simulink model "generator_library"  (R2019b)
settings: Solver=VariableStepAuto  StartTime=0.0  StopTime=10.0  RelTol=1e-3
undefined symbols (not defined in the file or in its folder): dataSim, dyn, Fnom, g, genTpd0, genTppd0, genTppq0, genTpq0, genXd, genXl, genXpd, genXppd, genXppq, genXpq, genXq, ifd, l, p, sys, vt
libraries: powerlib x27, simulink x10, powerlib_meascontrol x5, GenLib x2
settings Model: Creator=gdudgeon  LastModifiedBy=gdudgeon
settings SFSimCC: CustomCodeUndefinedFunction=UseInterfaceOnly

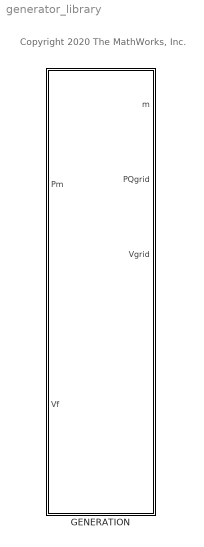
== system generator_library ==
  note: Copyright 2020 The MathWorks, Inc.
  GENERATION : Subsystem  VariantControlMode=Label  Variant=on  LabelModeActiveChoice=Variant2
      settings: AttributesFormatString=%<BlockChoice>

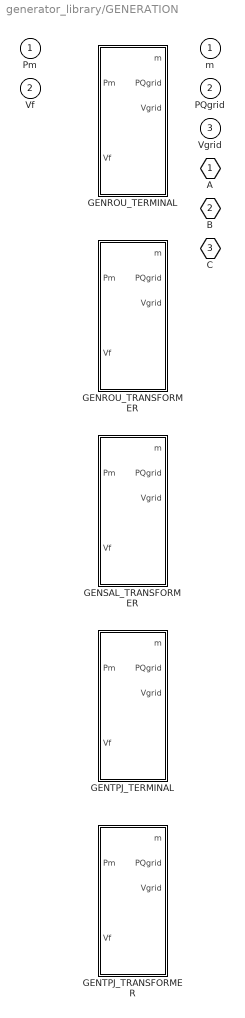
== system generator_library/GENERATION ==
  Pm : Inport
  Vf : Inport  Port=2
  GENROU_TERMINAL : Subsystem  VariantControl=Variant1  mask{g=sys.GENERATOR(1), p=dyn.genrou_31923_COLUSGT1}
      mask prompts: g "Generator Parameters"; p "Dynamic Parameters"
      mask DialogControl DescGroupVar Prompt: GENROU_TRANSFORMER
  GENROU_TRANSFORMER : Subsystem  VariantControl=Variant2  mask{g=sys.GENERATOR(2), t=sys.TRANSFORMER, p=dyn.genrou_102_GAS}
      mask prompts: g "Generator Parameters"; t "Transformer Parameters"; p "Dynamic Parameters"
      mask DialogControl DescGroupVar Prompt: GENROU_TRANSFORMER
  GENSAL_TRANSFORMER : Subsystem  VariantControl=Variant3  mask{g=sys.GENERATOR(2), t=sys.TRANSFORMER, p=dyn.gentpj_102_HYDRO}
      mask prompts: g "Generator Parameters"; t "Transformer Parameters"; p "Dynamic Parameters"
      mask DialogControl DescGroupVar Prompt: GENSAL_TRANSFORMER
  GENTPJ_TERMINAL : Subsystem  VariantControl=Variant4  mask{g=g, t=t, p=p}
      mask prompts: g "Generator Parameters"; t "Transformer Parameters"; p "Dynamic Parameters"
      mask DialogControl DescGroupVar Prompt: GENTPJ_TRANSFORMER
  GENTPJ_TRANSFORMER : Subsystem  VariantControl=Variant5  mask{g=sys.GENERATOR(2), t=sys.TRANSFORMER, p=dyn.gentpj_102_HYDRO}
      mask prompts: g "Generator Parameters"; t "Transformer Parameters"; p "Dynamic Parameters"
      mask DialogControl DescGroupVar Prompt: GENTPJ_TRANSFORMER
  A : PMIOPort  Side=Right
  B : PMIOPort  Port=2  Side=Right
  C : PMIOPort  Port=3  Side=Right
  m : Outport  VectorParamsAs1DForOutWhenUnconnected=off
  PQgrid : Outport  Port=2  VectorParamsAs1DForOutWhenUnconnected=off
  Vgrid : Outport  Port=3  VectorParamsAs1DForOutWhenUnconnected=off

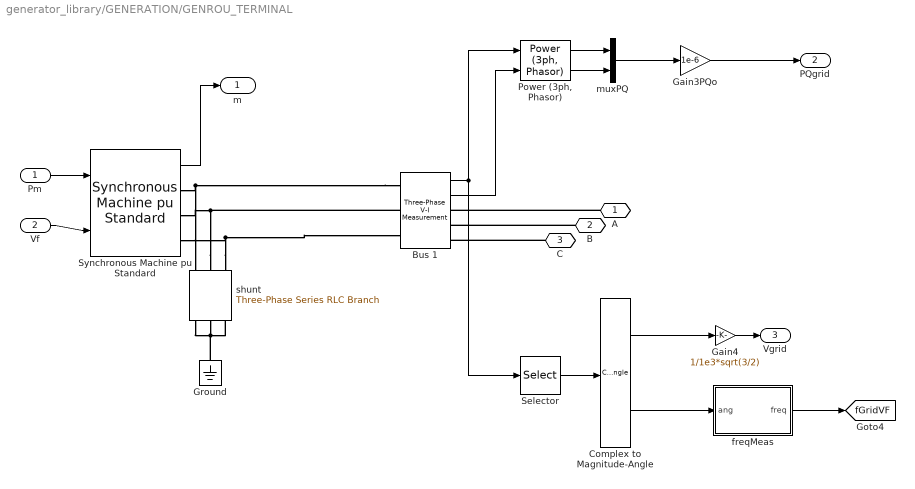
== system generator_library/GENERATION/GENROU_TERMINAL ==
  Pm : Inport
  Vf : Inport  Port=2
  Bus 1 : powerlib/Measurements/Three-Phase V-I Measurement  VoltageMeasurement=phase-to-ground  SetLabelV=off  LabelV=Vabc  Vpu=off  VpuLL=off  CurrentMeasurement=yes  SetLabelI=off  LabelI=Iabc  Ipu=off  Pbase=100e6  Vbase=500e3  OutputType=Complex  PhasorSimulation=on  PSBequivalent=0
      settings: SourceProductName=Simscape Electrical
  Complex to Magnitude-Angle : ComplexToMagnitudeAngle
  Gain3PQo : Gain  Gain=1e-6
  Gain4 : Gain  Gain=1/1e3*sqrt(3/2)
  Ground : powerlib/Elements/Ground  LConnTagsString=a
      settings: SourceProductName=Simscape Electrical
  "Power (3ph, Phasor)" : powerlib_meascontrol/Measurements/Power (3ph, Phasor)
      settings: SourceProductName=Simscape Electrical  SourceProductBaseCode=PS
  Selector : Selector  InputPortWidth=3  IndexOptions=Index vector (dialog)  Indices=1  OutputSizes=1
  Synchronous Machine pu Standard : powerlib/Machines/Synchronous Machine pu Standard  PresetModel=No  MechanicalLoad=Mechanical power Pm  ShowDetailedParameters=on  RotorType=Round  Units=per unit standard parameters  MeasurementBus=off  NominalParameters=[g.MBASE*1e6 g.BUSV*1e3 60]  Reactances1=[p.ld p.lpd p.lppd p.lq p.lpq p.lppd p.ll-0.01]  Reactances2=[ genXd genXpd genXppd genXq genXpq genXppq genXl]  dAxisTimeConstants=Open-circuit  qAxisTimeConstants=Open-circuit  TimeConstants1="[ 4.4849  0.0681  0.1  ]"  TimeConstants2=[p.tpdo p.tppdo p.tpqo p.tppqo]  TimeConstants3="[  4.49  0.0681  0.0513  ]"  TimeConstants4=[ 8.0, 0.03, 0.3371, 0.0295 ]  TimeConstants5=[ 1.01, 0.053, 0.1 ]  TimeConstants6=[ 1.3201, 0.023, 1.0, 0.07 ]  TimeConstants7=[genTpd0 genTppd0 genTpq0 genTppq0]  TimeConstants8=[genTpd0 genTppd0 genTpq0 genTppq0]  StatorResistance=p.ra  Mechanical=[p.h p.d 2]  PolePairs=2  InitialConditions=[0 -89.4885 0.00587296 0.00587296 0.00587296 0 -120 120 1.00004]  SetSaturation=on  Saturation=[ifd; vt]  LoadFlowParameters=[2 0 0 0 0]  TsPowergui=0  TsBlock=-1  IterativeModel=Trapezoidal non iterative  IterativeDiscreteModel=Trapezoidal non iterative  BusType=PV  Pref=0  Qref=0  Qmin=-inf  Qmax=inf  PLF=0  QLF=0
      settings: SourceProductName=Simscape Electrical
  freqMeas : Subsystem
  muxPQ : Mux  Inputs=2
  shunt : powerlib/Elements/Three-Phase Series RLC Branch  LConnTagsString=A|B|C  RConnTagsString=A|B|C  BranchType=R  Resistance=1e6  Inductance=0.0025  Capacitance=0  Measurements=None
      settings: SourceProductName=Simscape Electrical
  A : PMIOPort  Side=Right
  B : PMIOPort  Port=2  Side=Right
  C : PMIOPort  Port=3  Side=Right
  m : Outport  VectorParamsAs1DForOutWhenUnconnected=off
  PQgrid : Outport  Port=2  VectorParamsAs1DForOutWhenUnconnected=off
  Vgrid : Outport  Port=3  VectorParamsAs1DForOutWhenUnconnected=off
  tag scope: fGridVF=global
  wires:
  muxPQ/1 -> Gain3PQo/1
  Bus 1/1 -> Selector/1, "Power (3ph, Phasor)"/1
  Bus 1/2 -> "Power (3ph, Phasor)"/2
  "Power (3ph, Phasor)"/1 -> muxPQ/1
  Pm/1 -> Synchronous Machine pu Standard/1
  Complex to Magnitude-Angle/1 -> Gain4/1
  Vf/1 -> Synchronous Machine pu Standard/2
  Gain3PQo/1 -> PQgrid/1
  Gain4/1 -> Vgrid/1
  "Power (3ph, Phasor)"/2 -> muxPQ/2
  Synchronous Machine pu Standard/1 -> m/1
  Selector/1 -> Complex to Magnitude-Angle/1
  Complex to Magnitude-Angle/2 -> freqMeas/1(ang)
  freqMeas/1(freq) -> [fGridVF]
  connections:
  shunt/LConn3 -- Bus 1/LConn3 -- Synchronous Machine pu Standard/RConn3
  Bus 1/LConn1 -- shunt/LConn1 -- Synchronous Machine pu Standard/RConn1
  shunt/LConn2 -- Bus 1/LConn2 -- Synchronous Machine pu Standard/RConn2
  A/RConn1 -- Bus 1/RConn1
  B/RConn1 -- Bus 1/RConn2
  C/RConn1 -- Bus 1/RConn3
  shunt/RConn1 -- Ground/LConn1 -- shunt/RConn2 -- shunt/RConn3

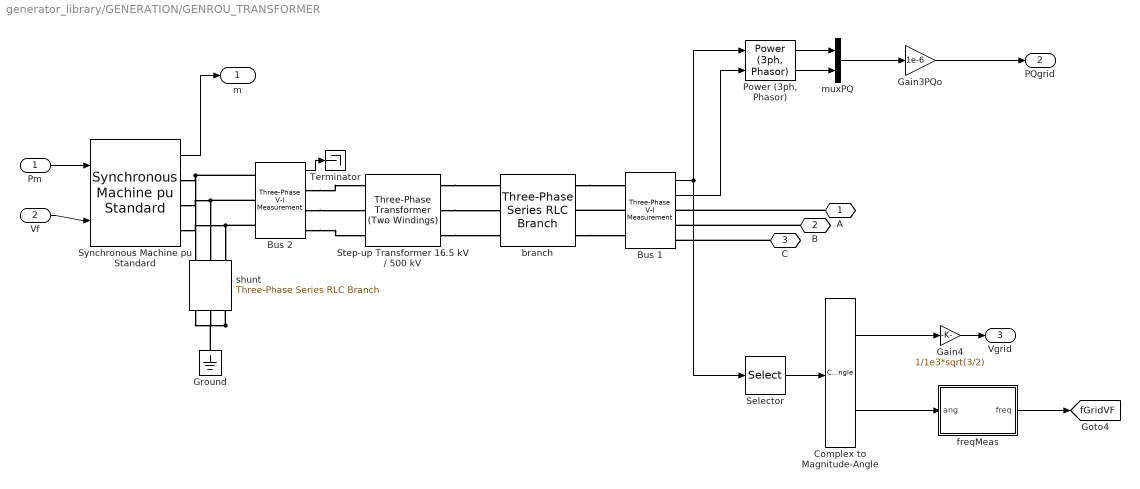
== system generator_library/GENERATION/GENROU_TRANSFORMER ==
  Pm : Inport
  Vf : Inport  Port=2
  Bus 1 : powerlib/Measurements/Three-Phase V-I Measurement  VoltageMeasurement=phase-to-ground  SetLabelV=off  LabelV=Vabc  Vpu=off  VpuLL=off  CurrentMeasurement=yes  SetLabelI=off  LabelI=Iabc  Ipu=off  Pbase=100e6  Vbase=500e3  OutputType=Complex  PhasorSimulation=on  PSBequivalent=0
      settings: SourceProductName=Simscape Electrical
  Bus 2 : powerlib/Measurements/Three-Phase V-I Measurement  VoltageMeasurement=phase-to-ground  SetLabelV=off  LabelV=Vabc  Vpu=off  VpuLL=off  CurrentMeasurement=no  SetLabelI=off  LabelI=Iabc  Ipu=off  Pbase=100e6  Vbase=500e3  OutputType=Complex  PhasorSimulation=on  PSBequivalent=0
      settings: SourceProductName=Simscape Electrical
  Complex to Magnitude-Angle : ComplexToMagnitudeAngle
  Gain3PQo : Gain  Gain=1e-6
  Gain4 : Gain  Gain=1/1e3*sqrt(3/2)
  Ground : powerlib/Elements/Ground  LConnTagsString=a
      settings: SourceProductName=Simscape Electrical
  "Power (3ph, Phasor)" : powerlib_meascontrol/Measurements/Power (3ph, Phasor)
      settings: SourceProductName=Simscape Electrical  SourceProductBaseCode=PS
  Selector : Selector  InputPortWidth=3  IndexOptions=Index vector (dialog)  Indices=1  OutputSizes=1
  Step-up Transformer 16.5 kV / 500 kV : powerlib/Elements/Three-Phase Transformer (Two Windings)  Winding1Connection=Yg  Winding2Connection=Yg  CoreType=Three single-phase transformers  SetSaturation=off  Hysteresis=off  DataFile='hysteresis'  SetInitialFlux=off  Measurements=None  UNITS=pu  NominalPower=[t.TBASE*1e6 60 ]  Winding1="[t.JV*1e3 t.PS_R/2  t.PS_X/2]"  Winding2="[t.IV*1e3 t.PS_R/2  t.PS_X/2]"  Rm=1/t.GMAG  Lm=1/abs(t.BMAG)  L0=0.5  Saturation="[ 0,0  ;  0.005,1.2  ;  1.0,1.4 ]"  InitialFluxes=[ 0.8 , -0.8 , 0.7 ]  BreakLoop=off  DiscreteSolver=Trapezoidal iterative  DataType=off  TransfoNumber=0
      settings: SourceProductName=Simscape Electrical
  Synchronous Machine pu Standard : powerlib/Machines/Synchronous Machine pu Standard  PresetModel=No  MechanicalLoad=Mechanical power Pm  ShowDetailedParameters=on  RotorType=Round  Units=per unit standard parameters  MeasurementBus=off  NominalParameters=[g.MBASE*1e6 g.BUSV*1e3 60]  Reactances1=[p.ld p.lpd p.lppd p.lq p.lpq p.lppd p.ll-0.01]  Reactances2=[ genXd genXpd genXppd genXq genXpq genXppq genXl]  dAxisTimeConstants=Open-circuit  qAxisTimeConstants=Open-circuit  TimeConstants1="[ 4.4849  0.0681  0.1  ]"  TimeConstants2=[p.tpdo p.tppdo p.tpqo p.tppqo]  TimeConstants3="[  4.49  0.0681  0.0513  ]"  TimeConstants4=[ 8.0, 0.03, 0.3371, 0.0295 ]  TimeConstants5=[ 1.01, 0.053, 0.1 ]  TimeConstants6=[ 1.3201, 0.023, 1.0, 0.07 ]  TimeConstants7=[genTpd0 genTppd0 genTpq0 genTppq0]  TimeConstants8=[genTpd0 genTppd0 genTpq0 genTppq0]  StatorResistance=p.ra  Mechanical=[p.h p.d 2]  PolePairs=2  InitialConditions=[0 -89.4885 0.00587296 0.00587296 0.00587296 0 -120 120 1.00004]  SetSaturation=on  Saturation=[ifd; vt]  LoadFlowParameters=[2 0 0 0 0]  TsPowergui=0  TsBlock=-1  IterativeModel=Trapezoidal non iterative  IterativeDiscreteModel=Trapezoidal non iterative  BusType=PV  Pref=0  Qref=0  Qmin=-inf  Qmax=inf  PLF=0  QLF=0
      settings: SourceProductName=Simscape Electrical
  Terminator : Terminator
  branch : powerlib/Elements/Three-Phase Series RLC Branch  LConnTagsString=A|B|C  RConnTagsString=A|B|C  BranchType=L  Resistance=0  Inductance=0.0003*500e3^2/100e6/2/pi/60  Capacitance=0  Measurements=None
      settings: SourceProductName=Simscape Electrical
  freqMeas : Subsystem
  muxPQ : Mux  Inputs=2
  shunt : powerlib/Elements/Three-Phase Series RLC Branch  LConnTagsString=A|B|C  RConnTagsString=A|B|C  BranchType=R  Resistance=1e6  Inductance=0.0025  Capacitance=0  Measurements=None
      settings: SourceProductName=Simscape Electrical
  A : PMIOPort  Side=Right
  B : PMIOPort  Port=2  Side=Right
  C : PMIOPort  Port=3  Side=Right
  m : Outport  VectorParamsAs1DForOutWhenUnconnected=off
  PQgrid : Outport  Port=2  VectorParamsAs1DForOutWhenUnconnected=off
  Vgrid : Outport  Port=3  VectorParamsAs1DForOutWhenUnconnected=off
  tag scope: fGridVF=global
  wires:
  freqMeas/1(freq) -> [fGridVF]
  Complex to Magnitude-Angle/2 -> freqMeas/1(ang)
  Selector/1 -> Complex to Magnitude-Angle/1
  Synchronous Machine pu Standard/1 -> m/1
  "Power (3ph, Phasor)"/2 -> muxPQ/2
  Gain4/1 -> Vgrid/1
  Gain3PQo/1 -> PQgrid/1
  Vf/1 -> Synchronous Machine pu Standard/2
  Complex to Magnitude-Angle/1 -> Gain4/1
  Pm/1 -> Synchronous Machine pu Standard/1
  "Power (3ph, Phasor)"/1 -> muxPQ/1
  Bus 1/2 -> "Power (3ph, Phasor)"/2
  Bus 1/1 -> "Power (3ph, Phasor)"/1, Selector/1
  muxPQ/1 -> Gain3PQo/1
  Bus 2/1 -> Terminator/1
  connections:
  Step-up Transformer 16.5 kV / 500 kV/RConn3 -- branch/LConn3
  Bus 1/LConn2 -- branch/RConn2
  shunt/RConn3 -- shunt/RConn2 -- Ground/LConn1 -- shunt/RConn1
  Step-up Transformer 16.5 kV / 500 kV/RConn2 -- branch/LConn2
  C/RConn1 -- Bus 1/RConn3
  branch/RConn1 -- Bus 1/LConn1
  branch/RConn3 -- Bus 1/LConn3
  B/RConn1 -- Bus 1/RConn2
  A/RConn1 -- Bus 1/RConn1
  Step-up Transformer 16.5 kV / 500 kV/RConn1 -- branch/LConn1
  Synchronous Machine pu Standard/RConn1 -- Bus 2/LConn1 -- shunt/LConn1
  Synchronous Machine pu Standard/RConn2 -- Bus 2/LConn2 -- shunt/LConn2
  Synchronous Machine pu Standard/RConn3 -- Bus 2/LConn3 -- shunt/LConn3
  Bus 2/RConn1 -- Step-up Transformer 16.5 kV / 500 kV/LConn1
  Bus 2/RConn2 -- Step-up Transformer 16.5 kV / 500 kV/LConn2
  Bus 2/RConn3 -- Step-up Transformer 16.5 kV / 500 kV/LConn3

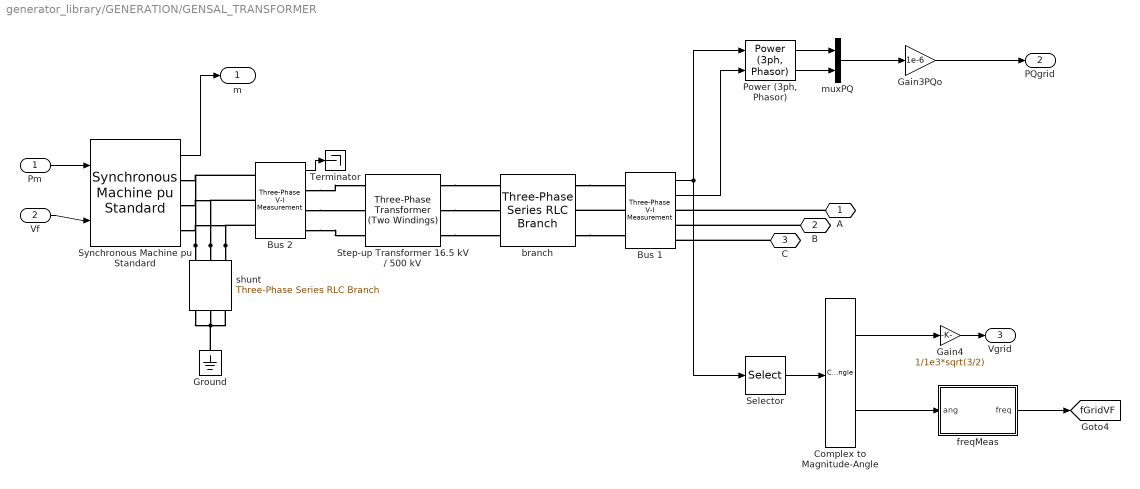
== system generator_library/GENERATION/GENSAL_TRANSFORMER ==
  Pm : Inport
  Vf : Inport  Port=2
  Bus 1 : powerlib/Measurements/Three-Phase V-I Measurement  VoltageMeasurement=phase-to-ground  SetLabelV=off  LabelV=Vabc  Vpu=off  VpuLL=off  CurrentMeasurement=yes  SetLabelI=off  LabelI=Iabc  Ipu=off  Pbase=100e6  Vbase=500e3  OutputType=Complex  PhasorSimulation=on  PSBequivalent=0
      settings: SourceProductName=Simscape Electrical
  Bus 2 : powerlib/Measurements/Three-Phase V-I Measurement  VoltageMeasurement=phase-to-ground  SetLabelV=off  LabelV=Vabc  Vpu=off  VpuLL=off  CurrentMeasurement=no  SetLabelI=off  LabelI=Iabc  Ipu=off  Pbase=100e6  Vbase=500e3  OutputType=Complex  PhasorSimulation=on  PSBequivalent=0
      settings: SourceProductName=Simscape Electrical
  Complex to Magnitude-Angle : ComplexToMagnitudeAngle
  Gain3PQo : Gain  Gain=1e-6
  Gain4 : Gain  Gain=1/1e3*sqrt(3/2)
  Ground : powerlib/Elements/Ground  LConnTagsString=a
      settings: SourceProductName=Simscape Electrical
  "Power (3ph, Phasor)" : powerlib_meascontrol/Measurements/Power (3ph, Phasor)
      settings: SourceProductName=Simscape Electrical  SourceProductBaseCode=PS
  Selector : Selector  InputPortWidth=3  IndexOptions=Index vector (dialog)  Indices=1  OutputSizes=1
  Step-up Transformer 16.5 kV / 500 kV : powerlib/Elements/Three-Phase Transformer (Two Windings)  Winding1Connection=Yg  Winding2Connection=Yg  CoreType=Three single-phase transformers  SetSaturation=off  Hysteresis=off  DataFile='hysteresis'  SetInitialFlux=off  Measurements=None  UNITS=pu  NominalPower=[t.TBASE*1e6 60 ]  Winding1="[t.JV*1e3 t.PS_R/2  t.PS_X/2]"  Winding2="[t.IV*1e3 t.PS_R/2  t.PS_X/2]"  Rm=1/t.GMAG  Lm=1/abs(t.BMAG)  L0=0.5  Saturation="[ 0,0  ;  0.005,1.2  ;  1.0,1.4 ]"  InitialFluxes=[ 0.8 , -0.8 , 0.7 ]  BreakLoop=off  DiscreteSolver=Trapezoidal iterative  DataType=off  TransfoNumber=0
      settings: SourceProductName=Simscape Electrical
  Synchronous Machine pu Standard : powerlib/Machines/Synchronous Machine pu Standard  PresetModel=No  MechanicalLoad=Mechanical power Pm  ShowDetailedParameters=on  RotorType=Salient-pole  Units=per unit standard parameters  MeasurementBus=off  NominalParameters=[g.MBASE*1e6 g.BUSV*1e3 60]  Reactances1=[p.ld p.lpd p.lppd p.lq p.lpq p.lppd p.ll-0.01]  Reactances2=[p.ld p.lpd p.lppd p.lq p.lppq p.ll]  dAxisTimeConstants=Open-circuit  qAxisTimeConstants=Open-circuit  TimeConstants1=[p.tpdo p.tppdo p.tppqo]  TimeConstants2=[p.tpdo p.tppdo p.tpqo p.tppqo]  TimeConstants3="[  4.49  0.0681  0.0513  ]"  TimeConstants4=[ 8.0, 0.03, 0.3371, 0.0295 ]  TimeConstants5=[ 1.01, 0.053, 0.1 ]  TimeConstants6=[ 1.3201, 0.023, 1.0, 0.07 ]  TimeConstants7=[genTpd0 genTppd0 genTpq0 genTppq0]  TimeConstants8=[genTpd0 genTppd0 genTpq0 genTppq0]  StatorResistance=p.ra  Mechanical=[p.h p.d 2]  PolePairs=2  InitialConditions=[0 -89.4885 0.00587296 0.00587296 0.00587296 0 -120 120 1.00004]  SetSaturation=on  Saturation=[ifd; vt]  LoadFlowParameters=[2 0 0 0 0]  TsPowergui=0  TsBlock=-1  IterativeModel=Trapezoidal non iterative  IterativeDiscreteModel=Trapezoidal non iterative  BusType=PV  Pref=0  Qref=0  Qmin=-inf  Qmax=inf  PLF=0  QLF=0
      settings: SourceProductName=Simscape Electrical
  Terminator : Terminator
  branch : powerlib/Elements/Three-Phase Series RLC Branch  LConnTagsString=A|B|C  RConnTagsString=A|B|C  BranchType=L  Resistance=0  Inductance=0.0003*500e3^2/100e6/2/pi/60  Capacitance=0  Measurements=None
      settings: SourceProductName=Simscape Electrical
  freqMeas : Subsystem
  muxPQ : Mux  Inputs=2
  shunt : powerlib/Elements/Three-Phase Series RLC Branch  LConnTagsString=A|B|C  RConnTagsString=A|B|C  BranchType=R  Resistance=1e6  Inductance=0.0025  Capacitance=0  Measurements=None
      settings: SourceProductName=Simscape Electrical
  A : PMIOPort  Side=Right
  B : PMIOPort  Port=2  Side=Right
  C : PMIOPort  Port=3  Side=Right
  m : Outport  VectorParamsAs1DForOutWhenUnconnected=off
  PQgrid : Outport  Port=2  VectorParamsAs1DForOutWhenUnconnected=off
  Vgrid : Outport  Port=3  VectorParamsAs1DForOutWhenUnconnected=off
  tag scope: fGridVF=global
  wires:
  Bus 2/1 -> Terminator/1
  muxPQ/1 -> Gain3PQo/1
  Bus 1/1 -> Selector/1, "Power (3ph, Phasor)"/1
  Bus 1/2 -> "Power (3ph, Phasor)"/2
  "Power (3ph, Phasor)"/1 -> muxPQ/1
  Pm/1 -> Synchronous Machine pu Standard/1
  Complex to Magnitude-Angle/1 -> Gain4/1
  Vf/1 -> Synchronous Machine pu Standard/2
  Gain3PQo/1 -> PQgrid/1
  Gain4/1 -> Vgrid/1
  "Power (3ph, Phasor)"/2 -> muxPQ/2
  Synchronous Machine pu Standard/1 -> m/1
  Selector/1 -> Complex to Magnitude-Angle/1
  Complex to Magnitude-Angle/2 -> freqMeas/1(ang)
  freqMeas/1(freq) -> [fGridVF]
  connections:
  Bus 2/RConn3 -- Step-up Transformer 16.5 kV / 500 kV/LConn3
  Bus 2/RConn2 -- Step-up Transformer 16.5 kV / 500 kV/LConn2
  Bus 2/RConn1 -- Step-up Transformer 16.5 kV / 500 kV/LConn1
  shunt/LConn3 -- Bus 2/LConn3 -- Synchronous Machine pu Standard/RConn3
  shunt/LConn2 -- Bus 2/LConn2 -- Synchronous Machine pu Standard/RConn2
  shunt/LConn1 -- Bus 2/LConn1 -- Synchronous Machine pu Standard/RConn1
  Step-up Transformer 16.5 kV / 500 kV/RConn1 -- branch/LConn1
  A/RConn1 -- Bus 1/RConn1
  B/RConn1 -- Bus 1/RConn2
  branch/RConn3 -- Bus 1/LConn3
  branch/RConn1 -- Bus 1/LConn1
  C/RConn1 -- Bus 1/RConn3
  Step-up Transformer 16.5 kV / 500 kV/RConn2 -- branch/LConn2
  shunt/RConn1 -- Ground/LConn1 -- shunt/RConn2 -- shunt/RConn3
  Bus 1/LConn2 -- branch/RConn2
  Step-up Transformer 16.5 kV / 500 kV/RConn3 -- branch/LConn3

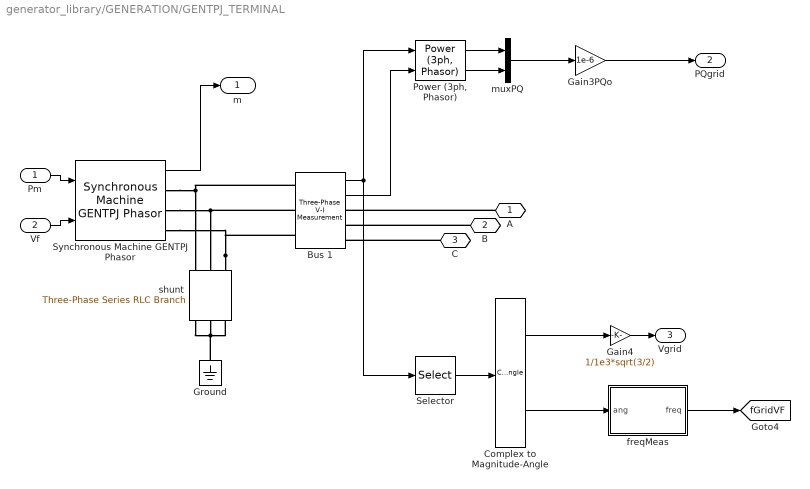
== system generator_library/GENERATION/GENTPJ_TERMINAL ==
  Pm : Inport
  Vf : Inport  Port=2
  Bus 1 : powerlib/Measurements/Three-Phase V-I Measurement  VoltageMeasurement=phase-to-ground  SetLabelV=off  LabelV=Vabc  Vpu=off  VpuLL=off  CurrentMeasurement=yes  SetLabelI=off  LabelI=Iabc  Ipu=off  Pbase=100e6  Vbase=500e3  OutputType=Complex  PhasorSimulation=on  PSBequivalent=0
      settings: SourceProductName=Simscape Electrical
  Complex to Magnitude-Angle : ComplexToMagnitudeAngle
  Gain3PQo : Gain  Gain=1e-6
  Gain4 : Gain  Gain=1/1e3*sqrt(3/2)
  Ground : powerlib/Elements/Ground  LConnTagsString=a
      settings: SourceProductName=Simscape Electrical
  "Power (3ph, Phasor)" : powerlib_meascontrol/Measurements/Power (3ph, Phasor)
      settings: SourceProductName=Simscape Electrical  SourceProductBaseCode=PS
  Selector : Selector  InputPortWidth=3  IndexOptions=Index vector (dialog)  Indices=1  OutputSizes=1
  Synchronous Machine GENTPJ Phasor : GenLib/Synchronous Machine GENTPJ Phasor  PresetModel=No  MechanicalLoad=Mechanical power Pm  ShowDetailedParameters=on  RotorType=Salient-pole  Units=per unit fundamental parameters  MeasurementBus=off  NominalParameters="[ 187E6  13800   60]"  Stator="[ 2.85E-03  0.114  1.19  0.36 ]"  Field="[ 5.79E-04  0.114]"  Dampers2=[0.0652, 0.5134, 0.0287, 0.2553, 7.765e-3, 0.9167 ]  Dampers1="[ 1.17E-02  0.182  1.97E-02  0.384 ]"  Mechanical=[ 3.7 0 20]  PolePairs=20  InitialConditions="[ 0  0  0  0  0  0  0  0  1 ]"  SetSaturation=off  Saturation=[0.6404,0.7127,0.8441,0.9214,0.9956,1.082,1.19,1.316,1.457;0.7,0.7698,0.8872,0.9466,0.9969,1.046,1.1,1.151,1.201]  LoadFlowParameters=[1,0,0,0,0]  TsPowergui=0  TsBlock=-1  IterativeModel=Trapezoidal non iterative  IterativeDiscreteModel=Trapezoidal non iterative  BusType=PV  Pref=0  Qref=0  Qmin=-inf  Qmax=inf  PLF=0  QLF=0  Pnom=g.MBASE*1e6  Vnom=g.BUSV*1e3  fnom=60  Ra=p.ra  Xl=p.ll  Xd=p.ld  Xq=p.lq  Xdp=p.lpd  Xqp=p.lpq  Xdpp=p.lppd  Xqpp=p.lppq  Tdop=p.tpdo  Tqop=p.tpqo  Tdopp=p.tppdo  Tqopp=p.tppqo  SatOption=Quadratic  Ifd=[0 0.5 0.6 0.7 0.8 0.9 1 1.0562 1.1184 1.1985 1.2994 1.4576 1.6524 2.2234]  Vag=[0 0.5 0.6 0.7 0.8 0.9 0.995 1.05 1.1 1.15 1.2 1.25 1.3 1.4]  S10S12=[p.s1 p.s12]  Kis=p.kis  SatOn=on  InputType=Mechanical power Pm  H=p.h  D=p.d
  freqMeas : Subsystem
  muxPQ : Mux  Inputs=2
  shunt : powerlib/Elements/Three-Phase Series RLC Branch  LConnTagsString=A|B|C  RConnTagsString=A|B|C  BranchType=R  Resistance=1e6  Inductance=0.0025  Capacitance=0  Measurements=None
      settings: SourceProductName=Simscape Electrical
  A : PMIOPort  Side=Right
  B : PMIOPort  Port=2  Side=Right
  C : PMIOPort  Port=3  Side=Right
  m : Outport  VectorParamsAs1DForOutWhenUnconnected=off
  PQgrid : Outport  Port=2  VectorParamsAs1DForOutWhenUnconnected=off
  Vgrid : Outport  Port=3  VectorParamsAs1DForOutWhenUnconnected=off
  tag scope: fGridVF=global
  wires:
  muxPQ/1 -> Gain3PQo/1
  Bus 1/1 -> Selector/1, "Power (3ph, Phasor)"/1
  Bus 1/2 -> "Power (3ph, Phasor)"/2
  "Power (3ph, Phasor)"/1 -> muxPQ/1
  Pm/1 -> Synchronous Machine GENTPJ Phasor/1
  Complex to Magnitude-Angle/1 -> Gain4/1
  Vf/1 -> Synchronous Machine GENTPJ Phasor/2
  Gain3PQo/1 -> PQgrid/1
  Gain4/1 -> Vgrid/1
  "Power (3ph, Phasor)"/2 -> muxPQ/2
  Synchronous Machine GENTPJ Phasor/1 -> m/1
  Selector/1 -> Complex to Magnitude-Angle/1
  Complex to Magnitude-Angle/2 -> freqMeas/1(ang)
  freqMeas/1(freq) -> [fGridVF]
  connections:
  shunt/LConn3 -- Synchronous Machine GENTPJ Phasor/RConn3 -- Bus 1/LConn3
  Bus 1/LConn2 -- Synchronous Machine GENTPJ Phasor/RConn2 -- shunt/LConn2
  Bus 1/LConn1 -- Synchronous Machine GENTPJ Phasor/RConn1 -- shunt/LConn1
  A/RConn1 -- Bus 1/RConn1
  B/RConn1 -- Bus 1/RConn2
  C/RConn1 -- Bus 1/RConn3
  shunt/RConn1 -- Ground/LConn1 -- shunt/RConn2 -- shunt/RConn3

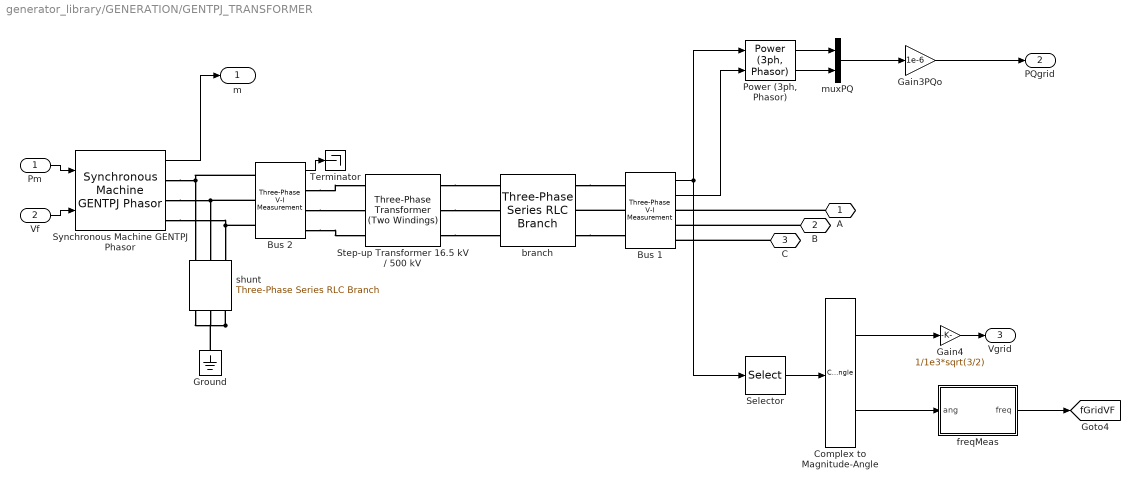
== system generator_library/GENERATION/GENTPJ_TRANSFORMER ==
  Pm : Inport
  Vf : Inport  Port=2
  Bus 1 : powerlib/Measurements/Three-Phase V-I Measurement  VoltageMeasurement=phase-to-ground  SetLabelV=off  LabelV=Vabc  Vpu=off  VpuLL=off  CurrentMeasurement=yes  SetLabelI=off  LabelI=Iabc  Ipu=off  Pbase=100e6  Vbase=500e3  OutputType=Complex  PhasorSimulation=on  PSBequivalent=0
      settings: SourceProductName=Simscape Electrical
  Bus 2 : powerlib/Measurements/Three-Phase V-I Measurement  VoltageMeasurement=phase-to-ground  SetLabelV=off  LabelV=Vabc  Vpu=off  VpuLL=off  CurrentMeasurement=no  SetLabelI=off  LabelI=Iabc  Ipu=off  Pbase=100e6  Vbase=500e3  OutputType=Complex  PhasorSimulation=on  PSBequivalent=0
      settings: SourceProductName=Simscape Electrical
  Complex to Magnitude-Angle : ComplexToMagnitudeAngle
  Gain3PQo : Gain  Gain=1e-6
  Gain4 : Gain  Gain=1/1e3*sqrt(3/2)
  Ground : powerlib/Elements/Ground  LConnTagsString=a
      settings: SourceProductName=Simscape Electrical
  "Power (3ph, Phasor)" : powerlib_meascontrol/Measurements/Power (3ph, Phasor)
      settings: SourceProductName=Simscape Electrical  SourceProductBaseCode=PS
  Selector : Selector  InputPortWidth=3  IndexOptions=Index vector (dialog)  Indices=1  OutputSizes=1
  Step-up Transformer 16.5 kV / 500 kV : powerlib/Elements/Three-Phase Transformer (Two Windings)  Winding1Connection=Yg  Winding2Connection=Yg  CoreType=Three single-phase transformers  SetSaturation=off  Hysteresis=off  DataFile='hysteresis'  SetInitialFlux=off  Measurements=None  UNITS=pu  NominalPower=[t.TBASE*1e6 60 ]  Winding1="[t.JV*1e3 t.PS_R/2  t.PS_X/2]"  Winding2="[t.IV*1e3 t.PS_R/2  t.PS_X/2]"  Rm=1/t.GMAG  Lm=1/abs(t.BMAG)  L0=0.5  Saturation="[ 0,0  ;  0.005,1.2  ;  1.0,1.4 ]"  InitialFluxes=[ 0.8 , -0.8 , 0.7 ]  BreakLoop=off  DiscreteSolver=Trapezoidal iterative  DataType=off  TransfoNumber=0
      settings: SourceProductName=Simscape Electrical
  Synchronous Machine GENTPJ Phasor : GenLib/Synchronous Machine GENTPJ Phasor  PresetModel=No  MechanicalLoad=Mechanical power Pm  ShowDetailedParameters=on  RotorType=Salient-pole  Units=per unit fundamental parameters  MeasurementBus=off  NominalParameters="[ 187E6  13800   60]"  Stator="[ 2.85E-03  0.114  1.19  0.36 ]"  Field="[ 5.79E-04  0.114]"  Dampers2=[0.0652, 0.5134, 0.0287, 0.2553, 7.765e-3, 0.9167 ]  Dampers1="[ 1.17E-02  0.182  1.97E-02  0.384 ]"  Mechanical=[ 3.7 0 20]  PolePairs=20  InitialConditions="[ 0  0  0  0  0  0  0  0  1 ]"  SetSaturation=off  Saturation=[0.6404,0.7127,0.8441,0.9214,0.9956,1.082,1.19,1.316,1.457;0.7,0.7698,0.8872,0.9466,0.9969,1.046,1.1,1.151,1.201]  LoadFlowParameters=[1,0,0,0,0]  TsPowergui=0  TsBlock=-1  IterativeModel=Trapezoidal non iterative  IterativeDiscreteModel=Trapezoidal non iterative  BusType=PV  Pref=0  Qref=0  Qmin=-inf  Qmax=inf  PLF=0  QLF=0  Pnom=g.MBASE*1e6  Vnom=g.BUSV*1e3  fnom=60  Ra=p.ra  Xl=p.ll  Xd=p.ld  Xq=p.lq  Xdp=p.lpd  Xqp=p.lpq  Xdpp=p.lppd  Xqpp=p.lppq  Tdop=p.tpdo  Tqop=p.tpqo  Tdopp=p.tppdo  Tqopp=p.tppqo  SatOption=Quadratic  Ifd=[0 0.5 0.6 0.7 0.8 0.9 1 1.0562 1.1184 1.1985 1.2994 1.4576 1.6524 2.2234]  Vag=[0 0.5 0.6 0.7 0.8 0.9 0.995 1.05 1.1 1.15 1.2 1.25 1.3 1.4]  S10S12=[p.s1 p.s12]  Kis=p.kis  SatOn=on  InputType=Mechanical power Pm  H=p.h  D=p.d
  Terminator : Terminator
  branch : powerlib/Elements/Three-Phase Series RLC Branch  LConnTagsString=A|B|C  RConnTagsString=A|B|C  BranchType=L  Resistance=0  Inductance=0.0003*500e3^2/100e6/2/pi/60  Capacitance=0  Measurements=None
      settings: SourceProductName=Simscape Electrical
  freqMeas : Subsystem
  muxPQ : Mux  Inputs=2
  shunt : powerlib/Elements/Three-Phase Series RLC Branch  LConnTagsString=A|B|C  RConnTagsString=A|B|C  BranchType=R  Resistance=1e6  Inductance=0.0025  Capacitance=0  Measurements=None
      settings: SourceProductName=Simscape Electrical
  A : PMIOPort  Side=Right
  B : PMIOPort  Port=2  Side=Right
  C : PMIOPort  Port=3  Side=Right
  m : Outport  VectorParamsAs1DForOutWhenUnconnected=off
  PQgrid : Outport  Port=2  VectorParamsAs1DForOutWhenUnconnected=off
  Vgrid : Outport  Port=3  VectorParamsAs1DForOutWhenUnconnected=off
  tag scope: fGridVF=global
  wires:
  freqMeas/1(freq) -> [fGridVF]
  Complex to Magnitude-Angle/2 -> freqMeas/1(ang)
  Selector/1 -> Complex to Magnitude-Angle/1
  Synchronous Machine GENTPJ Phasor/1 -> m/1
  "Power (3ph, Phasor)"/2 -> muxPQ/2
  Gain4/1 -> Vgrid/1
  Gain3PQo/1 -> PQgrid/1
  Vf/1 -> Synchronous Machine GENTPJ Phasor/2
  Complex to Magnitude-Angle/1 -> Gain4/1
  Pm/1 -> Synchronous Machine GENTPJ Phasor/1
  "Power (3ph, Phasor)"/1 -> muxPQ/1
  Bus 1/2 -> "Power (3ph, Phasor)"/2
  Bus 1/1 -> "Power (3ph, Phasor)"/1, Selector/1
  muxPQ/1 -> Gain3PQo/1
  Bus 2/1 -> Terminator/1
  connections:
  Step-up Transformer 16.5 kV / 500 kV/RConn3 -- branch/LConn3
  Bus 1/LConn2 -- branch/RConn2
  shunt/RConn3 -- shunt/RConn2 -- Ground/LConn1 -- shunt/RConn1
  Step-up Transformer 16.5 kV / 500 kV/RConn2 -- branch/LConn2
  C/RConn1 -- Bus 1/RConn3
  branch/RConn1 -- Bus 1/LConn1
  branch/RConn3 -- Bus 1/LConn3
  B/RConn1 -- Bus 1/RConn2
  A/RConn1 -- Bus 1/RConn1
  Step-up Transformer 16.5 kV / 500 kV/RConn1 -- branch/LConn1
  Bus 2/LConn1 -- Synchronous Machine GENTPJ Phasor/RConn1 -- shunt/LConn1
  Bus 2/LConn2 -- Synchronous Machine GENTPJ Phasor/RConn2 -- shunt/LConn2
  Bus 2/LConn3 -- Synchronous Machine GENTPJ Phasor/RConn3 -- shunt/LConn3
  Bus 2/RConn1 -- Step-up Transformer 16.5 kV / 500 kV/LConn1
  Bus 2/RConn2 -- Step-up Transformer 16.5 kV / 500 kV/LConn2
  Bus 2/RConn3 -- Step-up Transformer 16.5 kV / 500 kV/LConn3

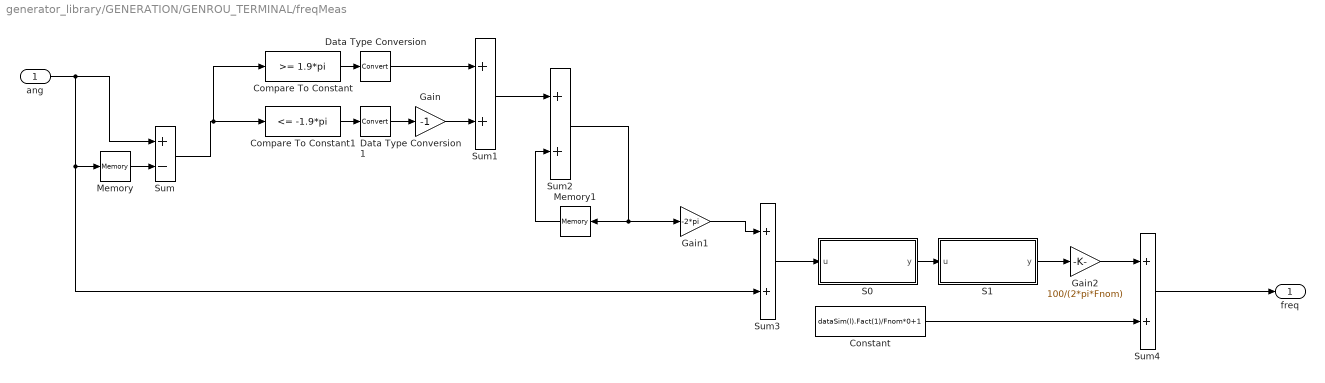
== system generator_library/GENERATION/GENROU_TERMINAL/freqMeas ==
  ang : Inport
  Compare To Constant : simulink/Logic and Bit Operations/Compare To Constant  relop=>=  const=1.9*pi  OutDataTypeStr=boolean
  Compare To Constant1 : simulink/Logic and Bit Operations/Compare To Constant  relop=<=  const=-1.9*pi  OutDataTypeStr=boolean
  Constant : Constant  Value=dataSim(l).Fact(1)/Fnom*0+1
  Data Type Conversion : DataTypeConversion
  Data Type Conversion1 : DataTypeConversion
  Gain : Gain  Gain=-1
  Gain1 : Gain  Gain=-2*pi
  Gain2 : Gain  Gain=100/(2*pi*Fnom)
  Memory : Memory  InheritSampleTime=on
  Memory1 : Memory  InheritSampleTime=on
  S0 : Subsystem
      mask Display: disp('s T_{w1} / (1 + s T_{w1})','texmode','on');
  S1 : Subsystem
      mask Display: disp('1/ (1 + s T)','texmode','on');
  Sum : Sum  Inputs=+-
  Sum{1..4} (4 alike) : Sum
  freq : Outport  VectorParamsAs1DForOutWhenUnconnected=off
  wires:
  Sum4/1 -> freq/1
  Gain2/1 -> Sum4/1
  Constant/1 -> Sum4/2
  Sum3/1 -> S0/1(u)
  Gain1/1 -> Sum3/1
  Data Type Conversion1/1 -> Gain/1
  Data Type Conversion/1 -> Sum1/1
  Memory/1 -> Sum/2
  Memory1/1 -> Sum2/2
  Gain/1 -> Sum1/2
  S0/1(y) -> S1/1(u)
  Compare To Constant/1 -> Data Type Conversion/1
  Compare To Constant1/1 -> Data Type Conversion1/1
  Sum2/1 -> Memory1/1, Gain1/1
  Sum/1 -> Compare To Constant1/1, Compare To Constant/1
  Sum1/1 -> Sum2/1
  ang/1 -> Sum3/2, Memory/1, Sum/1
  S1/1(y) -> Gain2/1

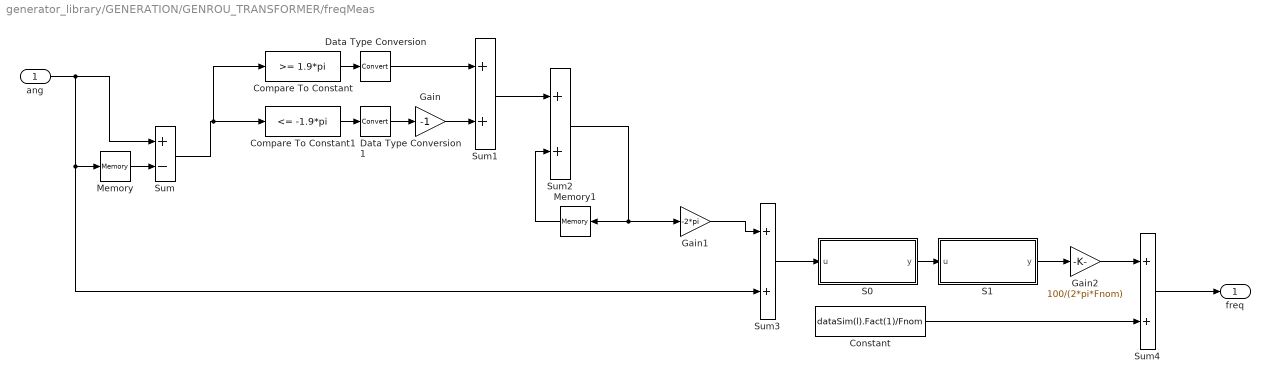
== system generator_library/GENERATION/GENROU_TRANSFORMER/freqMeas ==
  ang : Inport
  Compare To Constant : simulink/Logic and Bit Operations/Compare To Constant  relop=>=  const=1.9*pi  OutDataTypeStr=boolean
  Compare To Constant1 : simulink/Logic and Bit Operations/Compare To Constant  relop=<=  const=-1.9*pi  OutDataTypeStr=boolean
  Constant : Constant  Value=dataSim(l).Fact(1)/Fnom
  Data Type Conversion : DataTypeConversion
  Data Type Conversion1 : DataTypeConversion
  Gain : Gain  Gain=-1
  Gain1 : Gain  Gain=-2*pi
  Gain2 : Gain  Gain=100/(2*pi*Fnom)
  Memory : Memory  InheritSampleTime=on
  Memory1 : Memory  InheritSampleTime=on
  S0 : Subsystem
      mask Display: disp('s T_{w1} / (1 + s T_{w1})','texmode','on');
  S1 : Subsystem
      mask Display: disp('1/ (1 + s T)','texmode','on');
  Sum : Sum  Inputs=+-
  Sum{1..4} (4 alike) : Sum
  freq : Outport  VectorParamsAs1DForOutWhenUnconnected=off
  wires:
  S1/1(y) -> Gain2/1
  ang/1 -> Sum/1, Memory/1, Sum3/2
  Sum1/1 -> Sum2/1
  Sum/1 -> Compare To Constant/1, Compare To Constant1/1
  Sum2/1 -> Gain1/1, Memory1/1
  Compare To Constant1/1 -> Data Type Conversion1/1
  Compare To Constant/1 -> Data Type Conversion/1
  S0/1(y) -> S1/1(u)
  Gain/1 -> Sum1/2
  Memory1/1 -> Sum2/2
  Memory/1 -> Sum/2
  Data Type Conversion/1 -> Sum1/1
  Data Type Conversion1/1 -> Gain/1
  Gain1/1 -> Sum3/1
  Sum3/1 -> S0/1(u)
  Constant/1 -> Sum4/2
  Gain2/1 -> Sum4/1
  Sum4/1 -> freq/1

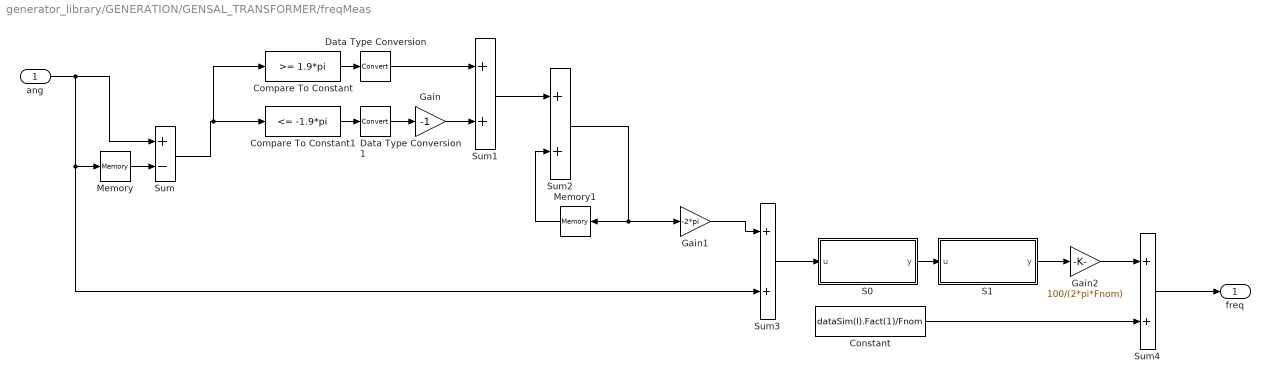
== system generator_library/GENERATION/GENSAL_TRANSFORMER/freqMeas ==
  ang : Inport
  Compare To Constant : simulink/Logic and Bit Operations/Compare To Constant  relop=>=  const=1.9*pi  OutDataTypeStr=boolean
  Compare To Constant1 : simulink/Logic and Bit Operations/Compare To Constant  relop=<=  const=-1.9*pi  OutDataTypeStr=boolean
  Constant : Constant  Value=dataSim(l).Fact(1)/Fnom
  Data Type Conversion : DataTypeConversion
  Data Type Conversion1 : DataTypeConversion
  Gain : Gain  Gain=-1
  Gain1 : Gain  Gain=-2*pi
  Gain2 : Gain  Gain=100/(2*pi*Fnom)
  Memory : Memory  InheritSampleTime=on
  Memory1 : Memory  InheritSampleTime=on
  S0 : Subsystem
      mask Display: disp('s T_{w1} / (1 + s T_{w1})','texmode','on');
  S1 : Subsystem
      mask Display: disp('1/ (1 + s T)','texmode','on');
  Sum : Sum  Inputs=+-
  Sum{1..4} (4 alike) : Sum
  freq : Outport  VectorParamsAs1DForOutWhenUnconnected=off
  wires:
  Sum4/1 -> freq/1
  Gain2/1 -> Sum4/1
  Constant/1 -> Sum4/2
  Sum3/1 -> S0/1(u)
  Gain1/1 -> Sum3/1
  Data Type Conversion1/1 -> Gain/1
  Data Type Conversion/1 -> Sum1/1
  Memory/1 -> Sum/2
  Memory1/1 -> Sum2/2
  Gain/1 -> Sum1/2
  S0/1(y) -> S1/1(u)
  Compare To Constant/1 -> Data Type Conversion/1
  Compare To Constant1/1 -> Data Type Conversion1/1
  Sum2/1 -> Memory1/1, Gain1/1
  Sum/1 -> Compare To Constant1/1, Compare To Constant/1
  Sum1/1 -> Sum2/1
  ang/1 -> Sum3/2, Memory/1, Sum/1
  S1/1(y) -> Gain2/1

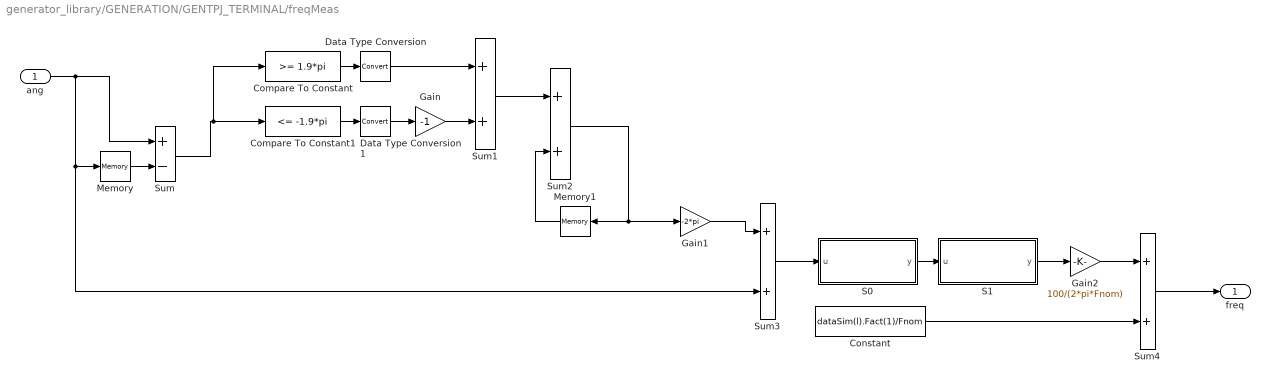
== system generator_library/GENERATION/GENTPJ_TERMINAL/freqMeas ==
  ang : Inport
  Compare To Constant : simulink/Logic and Bit Operations/Compare To Constant  relop=>=  const=1.9*pi  OutDataTypeStr=boolean
  Compare To Constant1 : simulink/Logic and Bit Operations/Compare To Constant  relop=<=  const=-1.9*pi  OutDataTypeStr=boolean
  Constant : Constant  Value=dataSim(l).Fact(1)/Fnom
  Data Type Conversion : DataTypeConversion
  Data Type Conversion1 : DataTypeConversion
  Gain : Gain  Gain=-1
  Gain1 : Gain  Gain=-2*pi
  Gain2 : Gain  Gain=100/(2*pi*Fnom)
  Memory : Memory  InheritSampleTime=on
  Memory1 : Memory  InheritSampleTime=on
  S0 : Subsystem
      mask Display: disp('s T_{w1} / (1 + s T_{w1})','texmode','on');
  S1 : Subsystem
      mask Display: disp('1/ (1 + s T)','texmode','on');
  Sum : Sum  Inputs=+-
  Sum{1..4} (4 alike) : Sum
  freq : Outport  VectorParamsAs1DForOutWhenUnconnected=off
  wires:
  Sum4/1 -> freq/1
  Gain2/1 -> Sum4/1
  Constant/1 -> Sum4/2
  Sum3/1 -> S0/1(u)
  Gain1/1 -> Sum3/1
  Data Type Conversion1/1 -> Gain/1
  Data Type Conversion/1 -> Sum1/1
  Memory/1 -> Sum/2
  Memory1/1 -> Sum2/2
  Gain/1 -> Sum1/2
  S0/1(y) -> S1/1(u)
  Compare To Constant/1 -> Data Type Conversion/1
  Compare To Constant1/1 -> Data Type Conversion1/1
  Sum2/1 -> Memory1/1, Gain1/1
  Sum/1 -> Compare To Constant1/1, Compare To Constant/1
  Sum1/1 -> Sum2/1
  ang/1 -> Sum3/2, Memory/1, Sum/1
  S1/1(y) -> Gain2/1

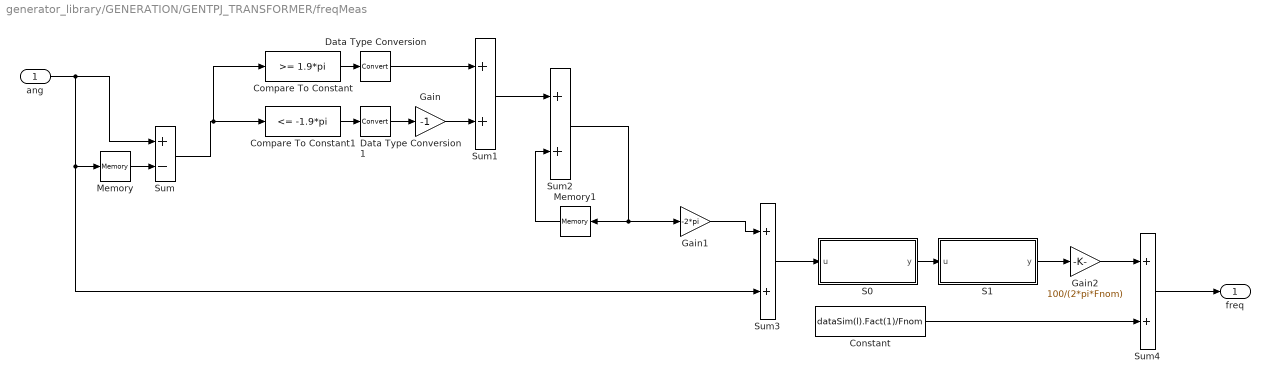
== system generator_library/GENERATION/GENTPJ_TRANSFORMER/freqMeas ==
  ang : Inport
  Compare To Constant : simulink/Logic and Bit Operations/Compare To Constant  relop=>=  const=1.9*pi  OutDataTypeStr=boolean
  Compare To Constant1 : simulink/Logic and Bit Operations/Compare To Constant  relop=<=  const=-1.9*pi  OutDataTypeStr=boolean
  Constant : Constant  Value=dataSim(l).Fact(1)/Fnom
  Data Type Conversion : DataTypeConversion
  Data Type Conversion1 : DataTypeConversion
  Gain : Gain  Gain=-1
  Gain1 : Gain  Gain=-2*pi
  Gain2 : Gain  Gain=100/(2*pi*Fnom)
  Memory : Memory  InheritSampleTime=on
  Memory1 : Memory  InheritSampleTime=on
  S0 : Subsystem
      mask Display: disp('s T_{w1} / (1 + s T_{w1})','texmode','on');
  S1 : Subsystem
      mask Display: disp('1/ (1 + s T)','texmode','on');
  Sum : Sum  Inputs=+-
  Sum{1..4} (4 alike) : Sum
  freq : Outport  VectorParamsAs1DForOutWhenUnconnected=off
  wires:
  S1/1(y) -> Gain2/1
  ang/1 -> Sum/1, Memory/1, Sum3/2
  Sum1/1 -> Sum2/1
  Sum/1 -> Compare To Constant/1, Compare To Constant1/1
  Sum2/1 -> Gain1/1, Memory1/1
  Compare To Constant1/1 -> Data Type Conversion1/1
  Compare To Constant/1 -> Data Type Conversion/1
  S0/1(y) -> S1/1(u)
  Gain/1 -> Sum1/2
  Memory1/1 -> Sum2/2
  Memory/1 -> Sum/2
  Data Type Conversion/1 -> Sum1/1
  Data Type Conversion1/1 -> Gain/1
  Gain1/1 -> Sum3/1
  Sum3/1 -> S0/1(u)
  Constant/1 -> Sum4/2
  Gain2/1 -> Sum4/1
  Sum4/1 -> freq/1

== system generator_library/GENERATION/GENROU_TERMINAL/freqMeas/S0 ==
  u : Inport
  Gain : Gain  Gain=1/1e-2
  Gain1 : Gain  Gain=1e-2
  Integrator : Integrator
  Sum : Sum  Inputs=|+-
  y : Outport  InitialOutput=0  VectorParamsAs1DForOutWhenUnconnected=off
  wires:
  Gain1/1 -> y/1
  Integrator/1 -> Sum/2
  Gain/1 -> Integrator/1, Gain1/1
  Sum/1 -> Gain/1
  u/1 -> Sum/1

== system generator_library/GENERATION/GENROU_TERMINAL/freqMeas/S1 ==
  u : Inport
  Gain2 : Gain  Gain=100
  Integrator1 : Integrator
  Sum : Sum  Inputs=|+-
  y : Outport  InitialOutput=0  VectorParamsAs1DForOutWhenUnconnected=off
  wires:
  u/1 -> Sum/1
  Sum/1 -> Gain2/1
  Integrator1/1 -> y/1, Sum/2
  Gain2/1 -> Integrator1/1

== system generator_library/GENERATION/GENROU_TRANSFORMER/freqMeas/S0 ==
  u : Inport
  Gain : Gain  Gain=1/1e-2
  Gain1 : Gain  Gain=1e-2
  Integrator : Integrator
  Sum : Sum  Inputs=|+-
  y : Outport  InitialOutput=0  VectorParamsAs1DForOutWhenUnconnected=off
  wires:
  u/1 -> Sum/1
  Sum/1 -> Gain/1
  Gain/1 -> Gain1/1, Integrator/1
  Integrator/1 -> Sum/2
  Gain1/1 -> y/1

== system generator_library/GENERATION/GENROU_TRANSFORMER/freqMeas/S1 ==
  u : Inport
  Gain2 : Gain  Gain=100
  Integrator1 : Integrator
  Sum : Sum  Inputs=|+-
  y : Outport  InitialOutput=0  VectorParamsAs1DForOutWhenUnconnected=off
  wires:
  Gain2/1 -> Integrator1/1
  Integrator1/1 -> Sum/2, y/1
  Sum/1 -> Gain2/1
  u/1 -> Sum/1

== system generator_library/GENERATION/GENSAL_TRANSFORMER/freqMeas/S0 ==
  u : Inport
  Gain : Gain  Gain=1/1e-2
  Gain1 : Gain  Gain=1e-2
  Integrator : Integrator
  Sum : Sum  Inputs=|+-
  y : Outport  InitialOutput=0  VectorParamsAs1DForOutWhenUnconnected=off
  wires:
  Gain1/1 -> y/1
  Integrator/1 -> Sum/2
  Gain/1 -> Integrator/1, Gain1/1
  Sum/1 -> Gain/1
  u/1 -> Sum/1

== system generator_library/GENERATION/GENSAL_TRANSFORMER/freqMeas/S1 ==
  u : Inport
  Gain2 : Gain  Gain=100
  Integrator1 : Integrator
  Sum : Sum  Inputs=|+-
  y : Outport  InitialOutput=0  VectorParamsAs1DForOutWhenUnconnected=off
  wires:
  u/1 -> Sum/1
  Sum/1 -> Gain2/1
  Integrator1/1 -> y/1, Sum/2
  Gain2/1 -> Integrator1/1

== system generator_library/GENERATION/GENTPJ_TERMINAL/freqMeas/S0 ==
  u : Inport
  Gain : Gain  Gain=1/1e-2
  Gain1 : Gain  Gain=1e-2
  Integrator : Integrator
  Sum : Sum  Inputs=|+-
  y : Outport  InitialOutput=0  VectorParamsAs1DForOutWhenUnconnected=off
  wires:
  Gain1/1 -> y/1
  Integrator/1 -> Sum/2
  Gain/1 -> Integrator/1, Gain1/1
  Sum/1 -> Gain/1
  u/1 -> Sum/1

== system generator_library/GENERATION/GENTPJ_TERMINAL/freqMeas/S1 ==
  u : Inport
  Gain2 : Gain  Gain=100
  Integrator1 : Integrator
  Sum : Sum  Inputs=|+-
  y : Outport  InitialOutput=0  VectorParamsAs1DForOutWhenUnconnected=off
  wires:
  u/1 -> Sum/1
  Sum/1 -> Gain2/1
  Integrator1/1 -> y/1, Sum/2
  Gain2/1 -> Integrator1/1

== system generator_library/GENERATION/GENTPJ_TRANSFORMER/freqMeas/S0 ==
  u : Inport
  Gain : Gain  Gain=1/1e-2
  Gain1 : Gain  Gain=1e-2
  Integrator : Integrator
  Sum : Sum  Inputs=|+-
  y : Outport  InitialOutput=0  VectorParamsAs1DForOutWhenUnconnected=off
  wires:
  u/1 -> Sum/1
  Sum/1 -> Gain/1
  Gain/1 -> Gain1/1, Integrator/1
  Integrator/1 -> Sum/2
  Gain1/1 -> y/1

== system generator_library/GENERATION/GENTPJ_TRANSFORMER/freqMeas/S1 ==
  u : Inport
  Gain2 : Gain  Gain=100
  Integrator1 : Integrator
  Sum : Sum  Inputs=|+-
  y : Outport  InitialOutput=0  VectorParamsAs1DForOutWhenUnconnected=off
  wires:
  Gain2/1 -> Integrator1/1
  Integrator1/1 -> Sum/2, y/1
  Sum/1 -> Gain2/1
  u/1 -> Sum/1
